simulink model "bicycle_sim"  (R2018b)
settings: Solver=VariableStepAuto  StartTime=0.0  StopTime=30  RelTol=1e-3
values from neighbouring files (symbols this model uses):
  theta0 = atan2(ppval(fnder(sy,1), 0), ppval(fnder(sx,1), 0))    [bicycle.m]
  x0 = xwp(1)    [bicycle.m]
  y0 = ywp(1)    [bicycle.m]
undefined symbols (not defined in the file or in its folder): breaks, xc, xdc, xddc, yc, ydc, yddc
libraries: simulink_extras x2, simulink x1
settings Model: Creator=olivier  LastModifiedBy=olivier
settings SolverCC: ZeroCrossAlgorithm=Adaptive
settings DebuggingCC: MaskedZcDiagnostic=none

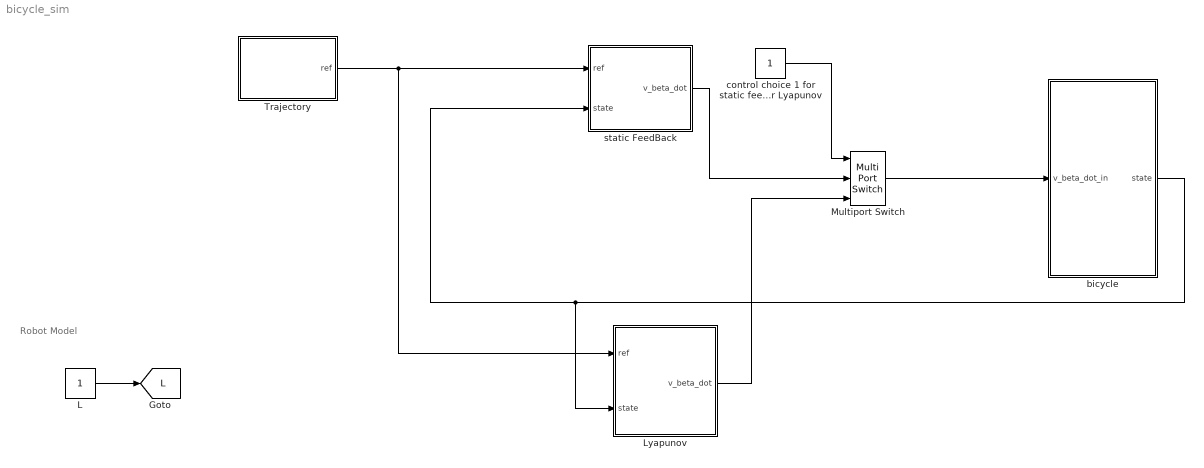
== system bicycle_sim ==
  note: Robot Model
  L : Constant
  Lyapunov : Subsystem
  Multiport Switch : MultiPortSwitch  Inputs=2
  Trajectory : Subsystem  TreatAsAtomicUnit=on
  bicycle : Subsystem  mask{L_error=0, radius_error=0, omega_max=100, beta_max=45, beta_dot_max=50}
      mask prompts: L_error "L error in percent"; radius_error "Radius error in percent"; omega_max "Max Rotation Velocity"; beta_max "Max Orientation"; beta_dot_max "Max Orientation Velocity"
  control choice 1 for static feedback 2 for Lyapunov : Constant
  static FeedBack : Subsystem
  tag scope: L=global
  wires:
  Lyapunov/1(v_beta_dot) -> Multiport Switch/3
  static FeedBack/1(v_beta_dot) -> Multiport Switch/2
  L/1 -> [L]
  Trajectory/1(ref) -> static FeedBack/1(ref), Lyapunov/1(ref)
  bicycle/1(state) -> Lyapunov/2(state), static FeedBack/2(state)
  control choice 1 for static feedback 2 for Lyapunov/1 -> Multiport Switch/1
  Multiport Switch/1 -> bicycle/1(v_beta_dot_in)

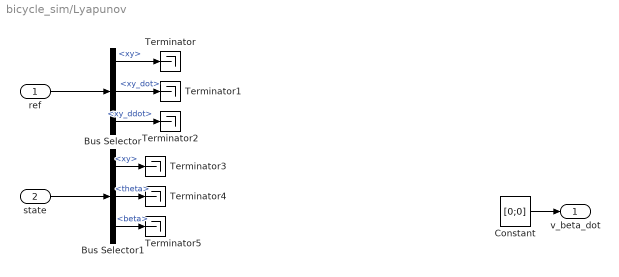
== system bicycle_sim/Lyapunov ==
  ref : Inport
  state : Inport  Port=2
  Bus Selector : BusSelector  OutputSignals=xy,xy_dot,xy_ddot
  Bus Selector1 : BusSelector  OutputSignals=xy,theta,beta
  Constant : Constant  Value=[0;0]
  Terminator{,1..5} (6 alike) : Terminator
  v_beta_dot : Outport
  wires:
  ref/1 -> Bus Selector/1
  state/1 -> Bus Selector1/1
  Bus Selector/1 -> Terminator/1  "<xy>"
  Bus Selector/2 -> Terminator1/1  "<xy_dot>"
  Bus Selector/3 -> Terminator2/1  "<xy_ddot>"
  Bus Selector1/3 -> Terminator5/1  "<beta>"
  Bus Selector1/2 -> Terminator4/1  "<theta>"
  Bus Selector1/1 -> Terminator3/1  "<xy>"
  Constant/1 -> v_beta_dot/1

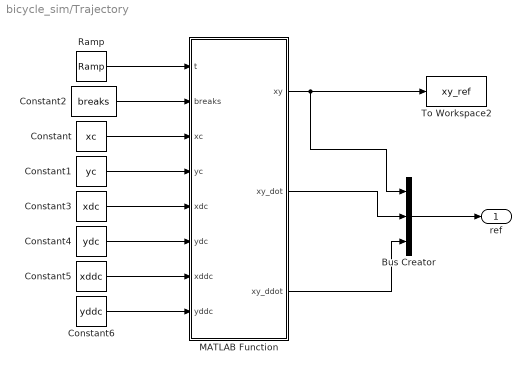
== system bicycle_sim/Trajectory ==
  Bus Creator : BusCreator  Inputs=3
  Constant : Constant  Value=xc  VectorParams1D=off
  Constant1 : Constant  Value=yc  VectorParams1D=off
  Constant2 : Constant  Value=breaks  VectorParams1D=off
  Constant3 : Constant  Value=xdc  VectorParams1D=off
  Constant4 : Constant  Value=ydc  VectorParams1D=off
  Constant5 : Constant  Value=xddc  VectorParams1D=off
  Constant6 : Constant  Value=yddc  VectorParams1D=off
  MATLAB Function : MATLAB Function  TreatAsAtomicUnit=on
  Ramp : simulink/Sources/Ramp  slope=1  start=0  InitialOutput=0
  To Workspace2 : ToWorkspace  VariableName=xy_ref  SampleTime=-1
      settings: Save2DSignal=2-D array (concatenate along first dimension)
  ref : Outport
  wires:
  Ramp/1 -> MATLAB Function/1(t)
  Constant3/1 -> MATLAB Function/5(xdc)
  Constant4/1 -> MATLAB Function/6(ydc)
  Constant/1 -> MATLAB Function/3(xc)
  Constant2/1 -> MATLAB Function/2(breaks)
  Constant1/1 -> MATLAB Function/4(yc)
  Constant5/1 -> MATLAB Function/7(xddc)
  Constant6/1 -> MATLAB Function/8(yddc)
  MATLAB Function/1(xy) -> Bus Creator/1, To Workspace2/1
  Bus Creator/1 -> ref/1
  MATLAB Function/3(xy_ddot) -> Bus Creator/3
  MATLAB Function/2(xy_dot) -> Bus Creator/2

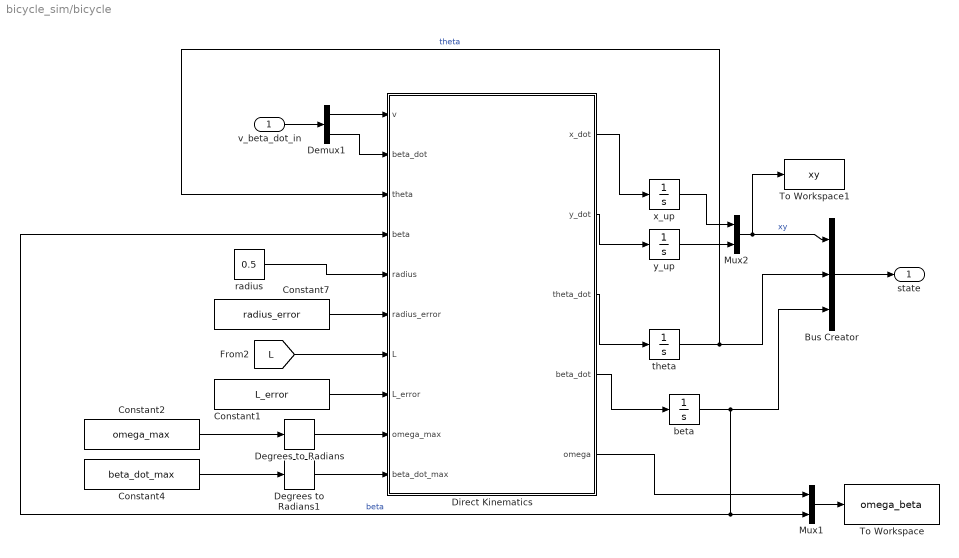
== system bicycle_sim/bicycle ==
  v_beta_dot_in : Inport
  Bus Creator : BusCreator  Inputs=3
  Constant1 : Constant  Value=L_error
  Constant2 : Constant  Value=omega_max
  Constant4 : Constant  Value=beta_dot_max
  Constant7 : Constant  Value=radius_error
  Degrees to Radians : simulink_extras/Transformations/Degrees to Radians
  Degrees to Radians1 : simulink_extras/Transformations/Degrees to Radians
  Demux1 : Demux  Outputs=2
  Direct Kinematics : MATLAB Function  TreatAsAtomicUnit=on
  Mux1 : Mux  Inputs=2
  Mux2 : Mux  Inputs=2
  To Workspace : ToWorkspace  VariableName=omega_beta  SampleTime=-1
      settings: Save2DSignal=2-D array (concatenate along first dimension)
  To Workspace1 : ToWorkspace  VariableName=xy  SampleTime=-1
      settings: Save2DSignal=2-D array (concatenate along first dimension)
  beta : Integrator  LimitOutput=on  UpperSaturationLimit=beta_max*pi/180  LowerSaturationLimit=-beta_max*pi/180
  radius : Constant  Value=0.5
  theta : Integrator  InitialCondition=theta0
  x_up : Integrator  InitialCondition=x0
  y_up : Integrator  InitialCondition=y0
  state : Outport
  wires:
  Direct Kinematics/2(y_dot) -> y_up/1
  Direct Kinematics/1(x_dot) -> x_up/1
  x_up/1 -> Mux2/1
  y_up/1 -> Mux2/2
  Mux2/1 -> Bus Creator/1, To Workspace1/1  "xy"
  Bus Creator/1 -> state/1
  v_beta_dot_in/1 -> Demux1/1
  Demux1/1 -> Direct Kinematics/1(v)
  [L] -> Direct Kinematics/7(L)
  Constant1/1 -> Direct Kinematics/8(L_error)
  Constant7/1 -> Direct Kinematics/6(radius_error)
  Direct Kinematics/3(theta_dot) -> theta/1
  Direct Kinematics/4(beta_dot) -> beta/1
  theta/1 -> Direct Kinematics/3(theta), Bus Creator/2  "theta"
  beta/1 -> Direct Kinematics/4(beta), Mux1/2, Bus Creator/3  "beta"
  Constant2/1 -> Degrees to Radians/1
  Constant4/1 -> Degrees to Radians1/1
  Direct Kinematics/5(omega) -> Mux1/1
  Mux1/1 -> To Workspace/1
  radius/1 -> Direct Kinematics/5(radius)
  Demux1/2 -> Direct Kinematics/2("beta_dot ")
  Degrees to Radians/1 -> Direct Kinematics/9(omega_max)
  Degrees to Radians1/1 -> Direct Kinematics/10(beta_dot_max)

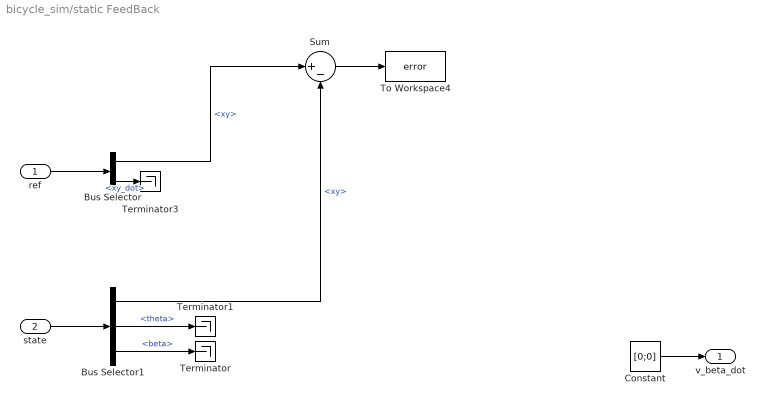
== system bicycle_sim/static FeedBack ==
  ref : Inport
  state : Inport  Port=2
  Bus Selector : BusSelector  OutputSignals=xy,xy_dot
  Bus Selector1 : BusSelector  OutputSignals=xy,theta,beta
  Constant : Constant  Value=[0;0]
  Sum : Sum  Inputs=|+-
  Terminator : Terminator
  Terminator1 : Terminator
  Terminator3 : Terminator
  To Workspace4 : ToWorkspace  VariableName=error  SampleTime=-1
      settings: Save2DSignal=2-D array (concatenate along first dimension)
  v_beta_dot : Outport
  wires:
  Sum/1 -> To Workspace4/1
  ref/1 -> Bus Selector/1
  state/1 -> Bus Selector1/1
  Bus Selector/1 -> Sum/1  "<xy>"
  Bus Selector1/3 -> Terminator/1  "<beta>"
  Bus Selector1/2 -> Terminator1/1  "<theta>"
  Bus Selector1/1 -> Sum/2  "<xy>"
  Bus Selector/2 -> Terminator3/1  "<xy_dot>"
  Constant/1 -> v_beta_dot/1

== matlab function bicycle_sim/bicycle/Direct Kinematics ==
  data: v input; beta_dot input; x_dot output; theta input; beta input; radius input; radius_error input; L input; L_error input; omega_max input; beta_dot_max input; y_dot output; theta_dot output; beta_dot output; omega output
function [x_dot, y_dot, theta_dot, beta_dot, omega]  = dk(v, beta_dot, theta, beta, radius, radius_error, L, L_error, omega_max, beta_dot_max)

% commanded wheel rotation velocity
omega = v/radius;
omega = max(-omega_max, min(omega, omega_max));

% actual linear velocity
v = (1+radius_error*0.01)*radius * omega;

% actual L value
L = (1+L_error*0.01)*L;

x_dot = v*cos(theta)*cos(beta);
y_dot = v*sin(theta)*cos(beta);
theta_dot = v*sin(beta)/L;
beta_dot = max(-beta_dot_max, min(beta_dot, beta_dot_max));

== matlab function bicycle_sim/Trajectory/MATLAB Function ==
  data: xy output; t input; breaks input; xc input; yc input; xy_dot output; xy_ddot output; xdc input; ydc input; xddc input; yddc input
function [xy, xy_dot, xy_ddot] = reference(t, breaks, xc, yc, xdc, ydc, xddc, yddc)

sx = mkpp(breaks, xc);
sy = mkpp(breaks, yc);


if t > sx.breaks(end)
    t = sx.breaks(end);
    xy_dot = [0; 0];
    xy_ddot = [0; 0];
else
    xy_dot = [ppval(mkpp(breaks, xdc), t); ppval(mkpp(breaks, ydc), t)];
    xy_ddot = [ppval(mkpp(breaks, xddc), t); ppval(mkpp(breaks, yddc), t)];
end
xy = [ppval(sx, t); ppval(sy, t)];
